simulink model "fft_tut"  (Simulink 4.00)
settings: Solver=FixedStepDiscrete  StartTime=0.0  StopTime=inf  RelTol=1e-3
PostLoadFcn:
  | set_param(gcs,'SimulationCommand','Update')
undefined symbols (not defined in the file or in its folder): get
libraries: dspxfrm3 x1, dspmtrx3 x1, dspsrcs3 x1, dspsnks3 x1
settings Model: RequirementInfo=9  LastModifiedBy=dfass  LimitDataPoints=off  ExtModeTrigMode=oneshot  ExtModeArmWhenConnect=off  BlockReductionOpt=off

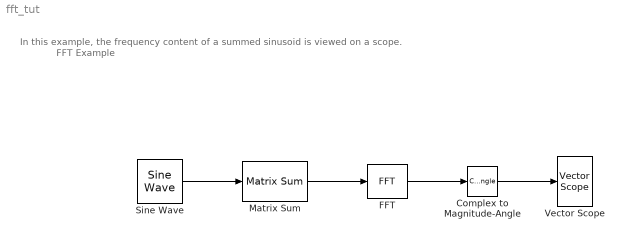
== system fft_tut ==
  note: FFT Example
  note: In this example, the frequency content of a summed sinusoid is viewed on a scope.
  Complex to Magnitude-Angle : ComplexToMagnitudeAngle  Output=Magnitude
  FFT : dspxfrm3/FFT
  Matrix Sum : dspmtrx3/Matrix Sum  Dim=Rows
  Sine Wave : dspsrcs3/Sine Wave  Amplitude=1  Frequency=[15 40]  Phase=0  SampleMode=Discrete  OutComplex=Real  CompMethod=Trigonometric Fcn  SampleTime=0.001  SamplesPerFrame=128  ResetState=Restart at time zero
  Vector Scope : dspsnks3/Vector Scope  ScopeProperties=off  Domain=Frequency  HorizSpan=1  DisplayProperties=off  AxisGrid=on  Memory=off  FrameNumber=on  AxisLegend=off  AxisZoom=off  OpenScopeAtSimStart=on  OpenScopeImmediately=off  FigPos=get(0,'defaultfigureposition')  AxisProperties=on  XUnits=Hertz  XRange=[0...Fs/2]  InheritXIncr=on  XIncr=1  XLabel=Samples  YUnits=Magnitude  YLabel=Amplitude  LineProperties=off
      settings: YMin=0.0723692553519949  YMax=69.3188381671759
  wires:
  Sine Wave/1 -> Matrix Sum/1
  Matrix Sum/1 -> FFT/1
  FFT/1 -> Complex to Magnitude-Angle/1
  Complex to Magnitude-Angle/1 -> Vector Scope/1
